simulink model "ShootingControlSystem"  (R2024b)
settings: Solver=VariableStepAuto  StartTime=0.0  StopTime=10.0  RelTol=1e-3
settings Model: Creator=Dell  LastModifiedBy=Dell

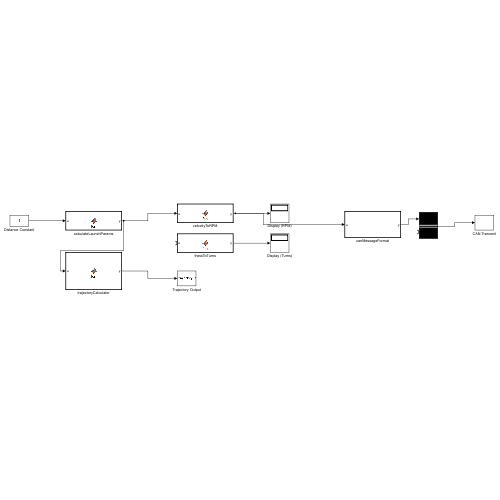
[thumbnail: Simulink's stored preview of the top-level diagram]
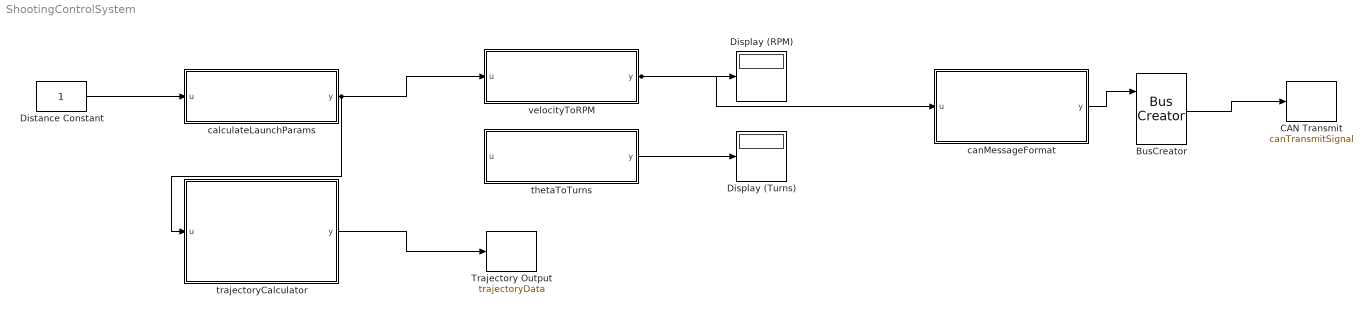
== system ShootingControlSystem ==
  BusCreator : BusCreator  Inputs=2
  CAN Transmit : ToWorkspace  VariableName=canTransmitSignal  SaveFormat=Timeseries  SampleTime=-1
  Display (RPM) : Display
  Display (Turns) : Display
  Distance Constant : Constant
  Trajectory Output : ToWorkspace  VariableName=trajectoryData  SaveFormat=Timeseries  SampleTime=-1
  calculateLaunchParams : MATLAB Function  TreatAsAtomicUnit=on
  canMessageFormat : MATLAB Function  TreatAsAtomicUnit=on
  thetaToTurns : MATLAB Function  TreatAsAtomicUnit=on
  trajectoryCalculator : MATLAB Function  TreatAsAtomicUnit=on
  velocityToRPM : MATLAB Function  TreatAsAtomicUnit=on
  wires:
  Distance Constant/1 -> calculateLaunchParams/1(u)
  calculateLaunchParams/1(y) -> velocityToRPM/1(u), trajectoryCalculator/1(u)
  velocityToRPM/1(y) -> Display (RPM)/1, canMessageFormat/1(u)
  thetaToTurns/1(y) -> Display (Turns)/1
  canMessageFormat/1(y) -> BusCreator/1
  BusCreator/1 -> CAN Transmit/1
  trajectoryCalculator/1(y) -> Trajectory Output/1

== matlab function ShootingControlSystem/calculateLaunchParams ==
  data: u input; y output
function y = fcn(u)

y = u;

== matlab function ShootingControlSystem/thetaToTurns ==
  data: u input; y output
function y = fcn(u)

y = u;

== matlab function ShootingControlSystem/canMessageFormat ==
  data: u input; y output
function y = fcn(u)

y = u;

== matlab function ShootingControlSystem/trajectoryCalculator ==
  data: u input; y output
function y = fcn(u)

y = u;

== matlab function ShootingControlSystem/velocityToRPM ==
  data: u input; y output
function y = fcn(u)

y = u;
